simulink model "rakett_sim"  (R2024a)
settings: Solver=VariableStepAuto  StartTime=0.0  StopTime=10.0  RelTol=1e-3
values from neighbouring files (symbols this model uses):
  g = 9.81    [rakett_init.m]
  k_l = (1/2) * ro * C_d * A    (= 0.0405988018623)    [rakett_init.m]
  m = 100    [rakett_init.m]
  r = [0 10000]    [rakett_init.m]
settings Model: Creator=Lars André  LastModifiedBy=Lars André

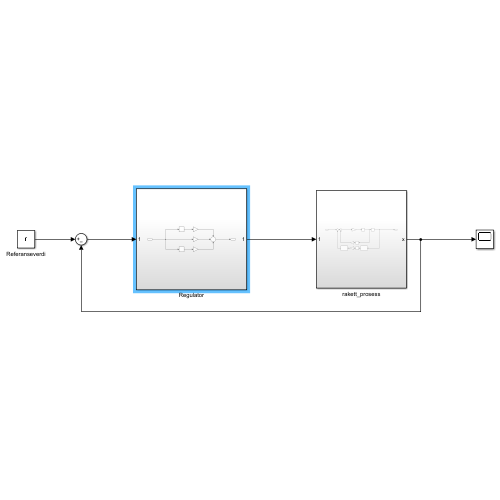
[thumbnail: Simulink's stored preview of the top-level diagram]
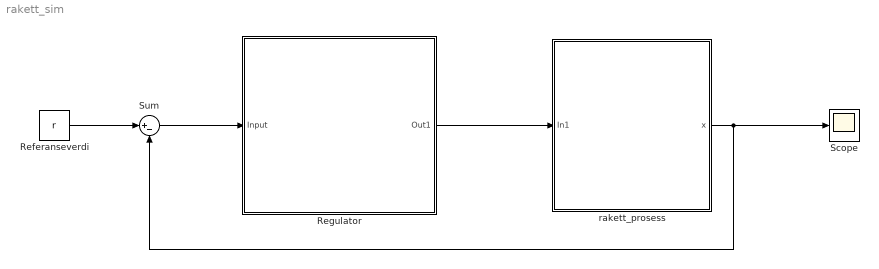
== system rakett_sim ==
  Referanseverdi : Constant  Value=r
  Regulator : Subsystem
  Scope : Scope
  Sum : Sum  Inputs=|+-
  rakett_prosess : Subsystem
  wires:
  rakett_prosess/1(x) -> Scope/1, Sum/2
  Regulator/1(Out1) -> rakett_prosess/1(In1)
  Referanseverdi/1 -> Sum/1
  Sum/1 -> Regulator/1(Input)

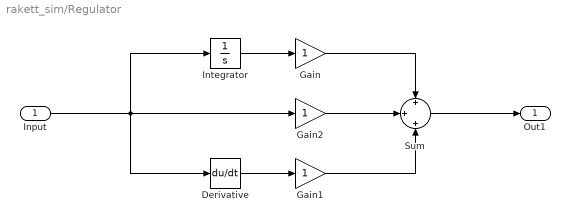
== system rakett_sim/Regulator ==
  Input : Inport
  Derivative : Derivative
  Gain : Gain
  Gain1 : Gain
  Gain2 : Gain
  Integrator : Integrator  InitialCondition=[0 0]
  Sum : Sum  Inputs=+|+|+
  Out1 : Outport
  wires:
  Input/1 -> Derivative/1, Integrator/1, Gain2/1
  Integrator/1 -> Gain/1
  Derivative/1 -> Gain1/1
  Gain1/1 -> Sum/3
  Gain2/1 -> Sum/2
  Gain/1 -> Sum/1
  Sum/1 -> Out1/1

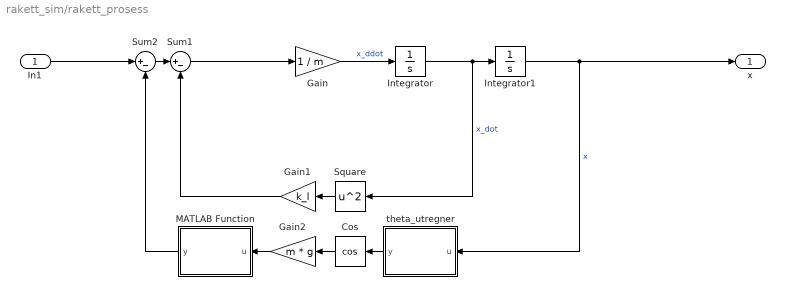
== system rakett_sim/rakett_prosess ==
  In1 : Inport
  Cos : Trigonometry  Operator=cos
  Gain : Gain  Gain=1 / m
  Gain1 : Gain  Gain=k_l
  Gain2 : Gain  Gain=m * g
  Integrator : Integrator
  Integrator1 : Integrator
  MATLAB Function : MATLAB Function  TreatAsAtomicUnit=on
  Square : Math  Operator=square
  Sum1 : Sum  Inputs=|+-
  Sum2 : Sum  Inputs=|+-
  theta_utregner : MATLAB Function  TreatAsAtomicUnit=on
  x : Outport
  wires:
  Gain1/1 -> Sum1/2
  Gain/1 -> Integrator/1  "x_ddot"
  Integrator/1 -> Square/1, Integrator1/1  "x_dot"
  Sum2/1 -> Sum1/1
  Square/1 -> Gain1/1
  In1/1 -> Sum2/1
  Sum1/1 -> Gain/1
  Integrator1/1 -> x/1, theta_utregner/1(u)  "x"
  Cos/1 -> Gain2/1
  theta_utregner/1(y) -> Cos/1
  Gain2/1 -> MATLAB Function/1(u)
  MATLAB Function/1(y) -> Sum2/2

== matlab function rakett_sim/rakett_prosess/theta_utregner ==
  data: u input; y output
function y = fcn(u)

y = atan(u(1) / u(2));

%Regner ut vinkel fra vektor der u[1] er x-retning og u[2] er y-retning

== matlab function rakett_sim/rakett_prosess/MATLAB Function ==
  data: u input; y output
function y = fcn(u)
y = [0 u];
